simulink model "vECUcontroller"  (R2024b)
settings: Solver=FixedStepAuto  StartTime=0.0  StopTime=3  FixedStep=0.001  RelTol=1e-3
model workspace (MAT data in the model file):
  Sig = Simulink.Signal
  Sig.Dimensions = -1
  Sig.DimensionsMode = 'auto'
  Sig.Complexity = 'auto'
  Sig.SampleTime = -1
  Sig.SamplingMode = 'auto'
  Sig.DataType = 'auto'
undefined symbols (not defined in the file): deinitSocket, fmuNum, portVal, stepSize
settings Model: Creator=hrkim  LastModifiedBy=hrkim
settings SFSimCC: SimCustomHeaderCode="#include \"../src/vECUwrapper.h\";"  SimUserSources=../src/vECUwrapper.c
settings RTWCC: RTWUseSimCustomCode=on  CustomHeaderCode="#include \"../src/vECUwrapper.h\";"  CustomSource=../src/vECUwrapper.c
settings CodeAppCC: MaxIdLength=255
settings GRTTargetCC: DynamicStringBufferSize=257

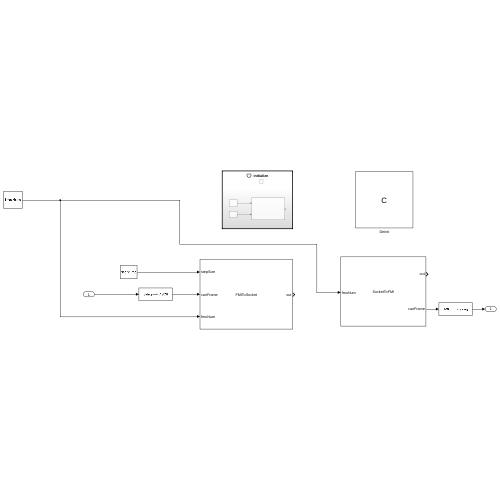
[thumbnail: Simulink's stored preview of the top-level diagram]
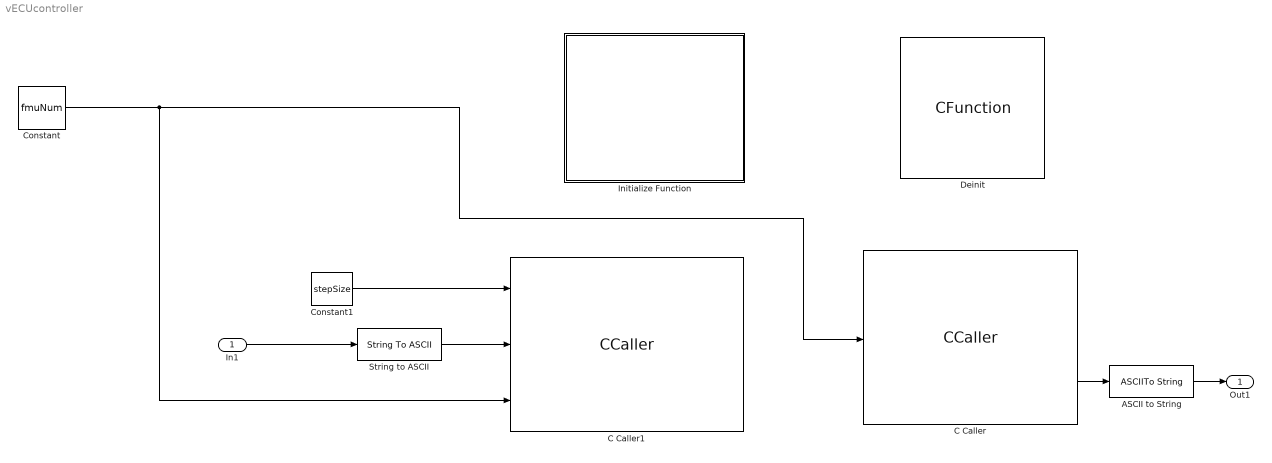
== system vECUcontroller ==
  In1 : Inport  OutDataTypeStr=string
  ASCII to String : ASCIIToString
  C Caller : CCaller  Priority=2  FunctionName=SocketToFMI  PortSpecificationStruct="%)30     .    > 4   8    (     @         %    \"     ,    !     0         %  0 \"0    $    _    07)G3F%M90  4&]R=$YA;64 4V-O<&4     26YD97@     5'EP90      4VEZ90      27-';&]B86P   X    P    !@    @    $          4    (     0    ,    !         !   P!O=70 #@   #     &    \"     0         !0    @    !     P    $         $  # &]U=  .    .     8    (    !          %    \"     $    &     0         0    !@   $]U='!U=   #@   #@    &    \"     8         !0    @    !     0    $         \"0    @               X    X    !@    @    $          4    (     0    4    !         !     %    :6YT,S(    .    ,     8    (    !          %    \"     $    !     0         0  $ ,0    X    P    !@    @    ) @        4    (     0    $    !          (  0      #@   #@    &    \"     0         !0    @    !    \"     $         $     @   !C86Y&<F%M90X    X    !@    @    $          4    (     0    @    !         !     (    8V%N1G)A;64.    .     8    (    !          %    \"     $    &     0         0    !@   $]U='!U=   #@   #@    &    \"     8         !0    @    !     0    $         \"0    @           #P/PX    X    !@    @    $          4    (     0    4    !         !     %    =6EN=#@    .    ,     8    (    !          %    \"     $    #     0         0  , ,C4U  X    P    !@    @    ) @        4    (     0    $    !          (  0      #@   #@    &    \"     0         !0    @    !    !@    $         $     8   !F;75.=6T   X    X    !@    @    $          4    (     0    8    !         !     &    9FUU3G5M   .    .     8    (    !          %    \"     $    %     0         0    !0   $EN<'5T    #@   #@    &    \"     8         !0    @    !     0    $         \"0    @               X    X    !@    @    $          4    (     0    4    !         !     %    :6YT,S(    .    ,     8    (    !          %    \"     $    !     0         0  $ ,0    X    P    !@    @    ) @        4    (     0    $    !          (  0"
  C Caller1 : CCaller  Priority=1  FunctionName=FMIToSocket  PortSpecificationStruct="%)30     .    * <   8    (     @         %    \"     0    !     0         %  0 \"0    $    _    07)G3F%M90  4&]R=$YA;64 4V-O<&4     26YD97@     5'EP90      4VEZ90      27-';&]B86P   X    P    !@    @    $          4    (     0    ,    !         !   P!O=70 #@   #     &    \"     0         !0    @    !     P    $         $  # &]U=  .    .     8    (    !          %    \"     $    &     0         0   ...(+2080 chars)"
  Constant : Constant  Value=fmuNum  OutDataTypeStr=int32
  Constant1 : Constant  Value=stepSize  OutDataTypeStr=double
  Deinit : CFunction  Priority=3  TerminateCode=deinitSocket();  CodegenTerminateCode=deinitSocket();  CustomCodeSettingLocation=ModelConfigurationParameters
  Initialize Function : Subsystem  TreatAsAtomicUnit=on
  String to ASCII : StringToASCII  OutputVectorSize=255
  Out1 : Outport  OutDataTypeStr=string
  wires:
  C Caller/2 -> ASCII to String/1
  Constant1/1 -> C Caller1/1
  In1/1 -> String to ASCII/1
  String to ASCII/1 -> C Caller1/2
  ASCII to String/1 -> Out1/1
  Constant/1 -> C Caller1/3, C Caller/1

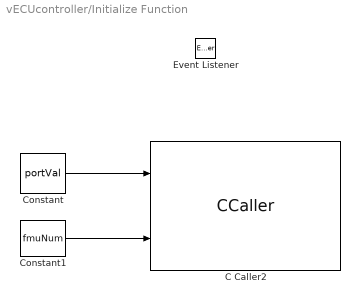
== system vECUcontroller/Initialize Function ==
  C Caller2 : CCaller  Priority=0  FunctionName=initSocket  PortSpecificationStruct="%)30     .    B 4   8    (     @         %    \"     ,    !     0         %  0 \"0    $    _    07)G3F%M90  4&]R=$YA;64 4V-O<&4     26YD97@     5'EP90      4VEZ90      27-';&]B86P   X    P    !@    @    $          4    (     0    ,    !         !   P!O=70 #@   #     &    \"     0         !0    @    !     P    $         $  # &]U=  .    .     8    (    !          %    \"     $    &     0         0    !@   $]U='!U=   #@   #@    &    \"     8         !0    @    !     0    $         \"0    @               X    X    !@    @    $          4    (     0    4    !         !     %    :6YT,S(    .    ,     8    (    !          %    \"     $    !     0         0  $ ,0    X    P    !@    @    ) @        4    (     0    $    !          (  0      #@   $     &    \"     0         !0    @    !    \"@    $         $     H   !P;W)T3G5M8F5R        #@   $     &    \"     0         !0    @    !    \"@    $         $     H   !P;W)T3G5M8F5R        #@   #@    &    \"     0         !0    @    !    !0    $         $     4   !);G!U=     X    X    !@    @    &          4    (     0    $    !          D    (               .    .     8    (    !          %    \"     $    %     0         0    !0   &EN=#,R    #@   #     &    \"     0         !0    @    !     0    $         $  ! #$    .    ,     8    (    \"0(        %    \"     $    !     0         \"  $       X    X    !@    @    $          4    (     0    8    !         !     &    9FUU3G5M   .    .     8    (    !          %    \"     $    &     0         0    !@   &9M=4YU;0  #@   #@    &    \"     0         !0    @    !    !0    $         $     4   !);G!U=     X    X    !@    @    &          4    (     0    $    !          D    (            \\#\\.    .     8    (    !          %    \"     $    %     0         0    !0   &EN=#,R    #@   #     &    \"     0         !0    @    !     0    $         $  ! #$    .    ,     8    (    \"0(        %    \"     $    !     0         \"  $"
  Constant : Constant  Value=portVal
  Constant1 : Constant  Value=fmuNum
  Event Listener : EventListener  DisableCoverage=on  EventName=reset
  wires:
  Constant/1 -> C Caller2/1
  Constant1/1 -> C Caller2/2
